simulink model "full_system_phase_control_dq0_discrete_quantized"  (R2015b)
settings: Solver=VariableStepAuto  StartTime=0.0  StopTime=6  FixedStep=1  RelTol=1e-2
values from neighbouring files (symbols this model uses):
  ad = cos(8*pi/256*n1+offset)    [Parameters.m]
  aq = -sin(8*pi/256*n1+offset)    [Parameters.m]
  bd = cos(8*pi/256*n1+offset-2/3*pi)    [Parameters.m]
  bq = -sin(8*pi/256*n1+offset-2/3*pi)    [Parameters.m]
  c_drag = -1/2*1.225*.804*.6    (= -0.29547)    [Parameters.m]
  cd = cos(8*pi/256*n1+offset+2/3*pi)    [Parameters.m]
  cq = -sin(8*pi/256*n1+offset+2/3*pi)    [Parameters.m]
  G1 = 12    [Parameters.m]
  G2 = 50    [Parameters.m]
  Ki = (3*alpha^2-((Kp*Kv)/(2*J_pro)-(Kv*R)/(J_pro*L)-(3*Kt^2)/(2*J_pro*L)))*L    (= 1.75664037993)    [Parameters.m]
  Kp = (3*alpha-Kv/J_pro-(R/(2*L)))*L    (= 0.0111498579282)    [Parameters.m]
  Kt = .07329    (= 0.07329)    [Parameters.m]
  L = 4e-5    (= 4e-05)    [Parameters.m]
  N = 4    [Parameters.m]
  n1 = 0:255    [Parameters.m]
  n2 = -1:.01:1    [Parameters.m]
  offset = 0    [Parameters.m]
  r = 11*.0254/2    (= 0.1397)    [Parameters.m]
  T = 1/10000    (= 0.0001)    [Parameters.m]
  third_phase = sin(3*asin(n2))    [Parameters.m]
undefined symbols (not defined in the file or in its folder): DiscIntNeverNeededParam, sigbuilder_block
libraries: fl_lib x19, nesl_utility x11, pe_lib x2, simulink x2, powerlib_meascontrol x1
settings Model: Creator=Martin Andersen  LastModifiedBy=Martin Andersen
settings SolverCC: AlgebraicLoopSolver=LineSearch

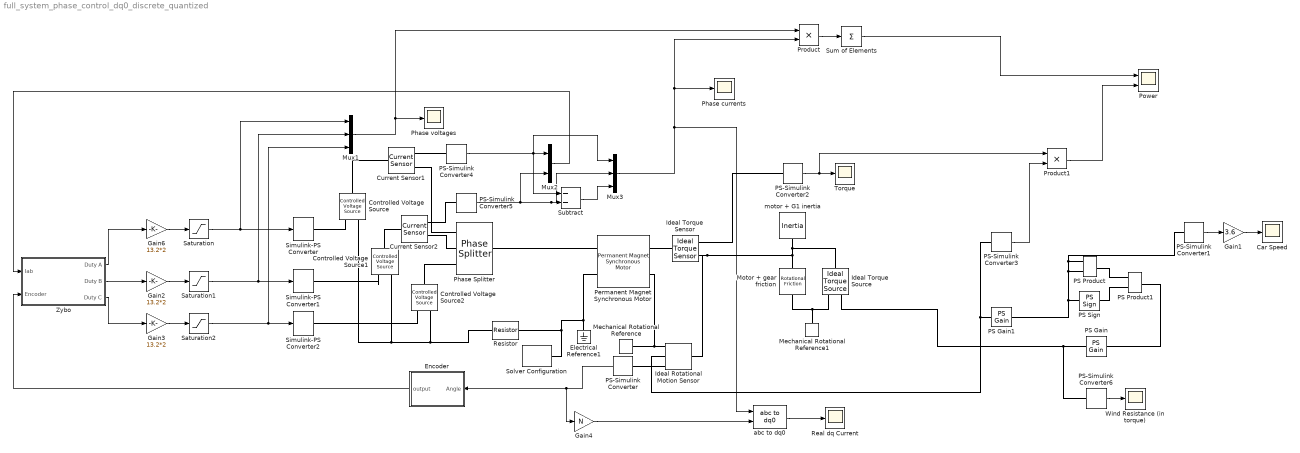
== system full_system_phase_control_dq0_discrete_quantized ==
  Car Speed : Scope
  Controlled Voltage Source : fl_lib/Electrical/Electrical Sources/Controlled Voltage Source
  Controlled Voltage Source1 : fl_lib/Electrical/Electrical Sources/Controlled Voltage Source
  Controlled Voltage Source2 : fl_lib/Electrical/Electrical Sources/Controlled Voltage Source
  Current Sensor1 : fl_lib/Electrical/Electrical Sensors/Current Sensor
  Current Sensor2 : fl_lib/Electrical/Electrical Sensors/Current Sensor
  Electrical Reference1 : fl_lib/Electrical/Electrical Elements/Electrical Reference
  Encoder : Subsystem
  Gain1 : Gain  Gain=3.6
  Gain2 : Gain  Gain=13.2*2
  Gain3 : Gain  Gain=13.2*2
  Gain4 : Gain  Gain=N
  Gain6 : Gain  Gain=13.2*2
  Ideal Rotational Motion Sensor : fl_lib/Mechanical/Mechanical Sensors/Ideal Rotational Motion Sensor  offset=0 rad
  Ideal Torque Sensor : fl_lib/Mechanical/Mechanical Sensors/Ideal Torque Sensor
  Ideal Torque Source : fl_lib/Mechanical/Mechanical Sources/Ideal Torque Source
  Mechanical Rotational Reference : fl_lib/Mechanical/Rotational Elements/Mechanical Rotational Reference
  Mechanical Rotational Reference1 : fl_lib/Mechanical/Rotational Elements/Mechanical Rotational Reference
  Motor + gear friction : fl_lib/Mechanical/Rotational Elements/Rotational Friction  brkwy_trq=.5 N*m  Col_trq=.2 N*m  visc_coef=0.0001 N*m/(rad/s)  trans_coef=10 s/rad  vel_thr=1e-4 rad/s  w_specify=off  w_priority=None  w=0 rad/s  t_specify=off  t_priority=None  t=0 N*m
  Mux1 : Mux  Inputs=3
  Mux2 : Mux  Inputs=2
  Mux3 : Mux  Inputs=3
  PS Gain : fl_lib/Physical Signals/Functions/PS Gain  gain=c_drag*G1/G2*r
  PS Gain1 : fl_lib/Physical Signals/Functions/PS Gain  gain=G1/G2*r
  PS Product : fl_lib/Physical Signals/Functions/PS Product
  PS Product1 : fl_lib/Physical Signals/Functions/PS Product
  PS Sign : fl_lib/Physical Signals/Nonlinear Operators/PS Sign
  PS-Simulink Converter{,1..6} (7 alike) : nesl_utility/PS-Simulink Converter  PhysicalDomain=network_engine_domain  SubClassName=ps_output  LeftPortType=input  RightPortType=output  PseudoPeriodic=off  Frequencies=[]  Unit=1  AffineConversion=off
  Permanent Magnet Synchronous Motor : pe_lib/Machines/Permanent Magnet Rotor/Permanent Magnet Synchronous Motor  nPolePairs=N  pm_flux_linkage=Kt/N Wb  stator_param=1  Ld=L H  Lq=L H  L0=L H  Ls=L H  Lm=0 H  Ms=L/10 H  Rs=R Ohm  initial_currents=[0, 0, 0] A  axes_param=2  angular_position0=0 rad  rotor_offset=- pi / 2 rad  shift_3ph=[nan, nan, nan] rad  sqrt2OverSqrt3=nan  oneOverSqrt2=nan  twoPiOver3=nan  Lmin=1e-9 H
  Phase Splitter : pe_lib/Connections/Phase Splitter
  Phase currents : Scope
  Phase voltages : Scope
  Power : Scope  NumInputPorts=2
  Product : Product
  Product1 : Product
  Real dq Current : Scope
  Resistor : fl_lib/Electrical/Electrical Elements/Resistor  R=1e9 Ohm  i_specify=off  i_priority=None  i=0 A  v_specify=off  v_priority=None  v=0 V
  Saturation : Saturate  UpperLimit=13.2*2  LowerLimit=-13.2*2
  Saturation1 : Saturate  UpperLimit=13.2*2  LowerLimit=-13.2*2
  Saturation2 : Saturate  UpperLimit=13.2*2  LowerLimit=-13.2*2
  Simulink-PS Converter : nesl_utility/Simulink-PS Converter  PhysicalDomain=network_engine_domain  SubClassName=ps_input  LeftPortType=input  RightPortType=output  PseudoPeriodic=off  Frequencies=[]  NoiseDistribution=none  NoiseParameters=[]  Unit=1  AffineConversion=off  InputFiltering=off  SimscapeFilterOrder=1  InputFilterTimeConstant=0.001  UdotUserProvided=1
  Simulink-PS Converter1 : nesl_utility/Simulink-PS Converter  PhysicalDomain=network_engine_domain  SubClassName=ps_input  LeftPortType=input  RightPortType=output  PseudoPeriodic=off  Frequencies=[]  NoiseDistribution=none  NoiseParameters=[]  Unit=1  AffineConversion=off  InputFiltering=off  SimscapeFilterOrder=1  InputFilterTimeConstant=0.001  UdotUserProvided=1
  Simulink-PS Converter2 : nesl_utility/Simulink-PS Converter  PhysicalDomain=network_engine_domain  SubClassName=ps_input  LeftPortType=input  RightPortType=output  PseudoPeriodic=off  Frequencies=[]  NoiseDistribution=none  NoiseParameters=[]  Unit=1  AffineConversion=off  InputFiltering=off  SimscapeFilterOrder=1  InputFilterTimeConstant=0.001  UdotUserProvided=1
  Solver Configuration : nesl_utility/Solver Configuration  PhysicalDomain=network_engine_domain  SubClassName=solver  LeftPortType=input  RightPortType=generic  Accelerate=off  Tones=[]  Harmonics=[]  SimulateNoise=off  Profile=off  UseLocalSampling=off  EnableSwitchedLinearOptims=on  FrequencyDomain=off  UseCCode=off  RelTol=0.001  AbsTol=1e-06  MinStep=1e-09  ToWorkspace=off  RevertToSquareIcSolve=off  NumHomotopyIterations=100  PhasorMode=off  PhasorModeNumHarmonics=1  DoDC=off  ResidualTolerance=1e-09  UseLocalSolver=off  LocalSolverChoice=NE_BACKWARD_EULER_ADVANCER  LocalSolverSampleTime=0.001  DoFixedCost=off  MaxNonlinIter=3  MaxModeIter=2  LinearAlgebra=Sparse  DelaysMemoryBudget=1024  AutomaticFiltering=on  FilteringTimeConstant=0.001
  Subtract : Sum  Inputs=--
  Sum of Elements : Sum  Inputs=+
  Torque : Scope
  Wind Resistance (in torque) : Scope
  Zybo : Subsystem
  abc to dq0 : powerlib_meascontrol/Transformations/abc to dq0  Alignment=Aligned with phase A axis
  motor + G1 inertia : fl_lib/Mechanical/Rotational Elements/Inertia  inertia=J_pro kg*m^2  w_specify=off  w_priority=None  w=0 rad/s  t_specify=off  t_priority=None  t=0 N*m
  wires:
  PS-Simulink Converter1/1 -> Gain1/1
  Gain1/1 -> Car Speed/1
  PS-Simulink Converter4/1 -> Subtract/1, Mux3/1, Mux2/1
  PS-Simulink Converter5/1 -> Mux3/2, Subtract/2, Mux2/2
  PS-Simulink Converter6/1 -> Wind Resistance (in torque)/1
  Mux1/1 -> Product/1, Phase voltages/1
  Mux2/1 -> Zybo/1(Iab)
  PS-Simulink Converter2/1 -> Product1/1, Torque/1
  Product/1 -> Sum of Elements/1
  Sum of Elements/1 -> Power/1
  PS-Simulink Converter3/1 -> Product1/2
  Product1/1 -> Power/2
  Zybo/1(Duty A) -> Gain6/1
  PS-Simulink Converter/1 -> Gain4/1, Encoder/1(Angle)
  Encoder/1(output) -> Zybo/2(Encoder)
  Gain6/1 -> Saturation/1
  Gain2/1 -> Saturation1/1
  Gain3/1 -> Saturation2/1
  Saturation/1 -> Mux1/1, Simulink-PS Converter/1
  Saturation1/1 -> Mux1/2, Simulink-PS Converter1/1
  Zybo/2(Duty B) -> Gain2/1
  Zybo/3(Duty C) -> Gain3/1
  Saturation2/1 -> Mux1/3, Simulink-PS Converter2/1
  Subtract/1 -> Mux3/3
  Mux3/1 -> abc to dq0/1, Phase currents/1, Product/2
  Gain4/1 -> abc to dq0/2
  abc to dq0/1 -> Real dq Current/1
  connections:
  Permanent Magnet Synchronous Motor/LConn2 -- Resistor/RConn1 -- Solver Configuration/RConn1 -- Electrical Reference1/LConn1
  Ideal Rotational Motion Sensor/RConn1 -- Mechanical Rotational Reference/LConn1 -- Permanent Magnet Synchronous Motor/RConn2
  PS Sign/LConn1 -- PS-Simulink Converter1/LConn1 -- PS Product/LConn1 -- PS Product/LConn2 -- PS Gain1/RConn1
  PS Product1/LConn2 -- PS Sign/RConn1
  PS Product1/LConn1 -- PS Product/RConn1
  PS Gain/LConn1 -- PS Product1/RConn1
  PS-Simulink Converter6/LConn1 -- Ideal Torque Source/RConn1 -- PS Gain/RConn1
  PS-Simulink Converter/LConn1 -- Ideal Rotational Motion Sensor/RConn3
  Controlled Voltage Source/RConn1 -- Simulink-PS Converter/RConn1
  Controlled Voltage Source1/RConn1 -- Simulink-PS Converter1/RConn1
  Controlled Voltage Source2/RConn1 -- Simulink-PS Converter2/RConn1
  Controlled Voltage Source2/LConn1 -- Phase Splitter/RConn3
  Controlled Voltage Source1/RConn2 -- Controlled Voltage Source/RConn2 -- Resistor/LConn1 -- Controlled Voltage Source2/RConn2
  Phase Splitter/LConn1 -- Permanent Magnet Synchronous Motor/LConn1
  Current Sensor1/LConn1 -- Controlled Voltage Source/LConn1
  Current Sensor1/RConn2 -- Phase Splitter/RConn1
  Current Sensor2/LConn1 -- Controlled Voltage Source1/LConn1
  Current Sensor2/RConn2 -- Phase Splitter/RConn2
  PS-Simulink Converter4/LConn1 -- Current Sensor1/RConn1
  Current Sensor2/RConn1 -- PS-Simulink Converter5/LConn1
  Mechanical Rotational Reference1/LConn1 -- Ideal Torque Source/RConn2 -- Motor + gear friction/RConn1
  PS Gain1/LConn1 -- Ideal Rotational Motion Sensor/RConn2 -- PS-Simulink Converter3/LConn1
  motor + G1 inertia/LConn1 -- Ideal Rotational Motion Sensor/LConn1 -- Ideal Torque Sensor/RConn1 -- Motor + gear friction/LConn1 -- Ideal Torque Source/LConn1
  PS-Simulink Converter2/LConn1 -- Ideal Torque Sensor/RConn2
  Ideal Torque Sensor/LConn1 -- Permanent Magnet Synchronous Motor/RConn1

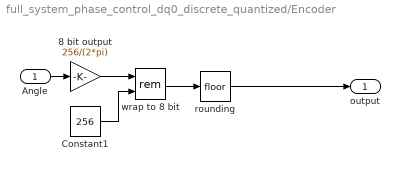
== system full_system_phase_control_dq0_discrete_quantized/Encoder ==
  Angle : Inport
  8 bit output : Gain  Gain=256/(2*pi)
  Constant1 : Constant  Value=256
  rounding : Rounding
  wrap to 8 bit : Math  Operator=rem  SaturateOnIntegerOverflow=on
  output : Outport
  wires:
  wrap to 8 bit/1 -> rounding/1
  Constant1/1 -> wrap to 8 bit/2
  8 bit output/1 -> wrap to 8 bit/1
  Angle/1 -> 8 bit output/1
  rounding/1 -> output/1

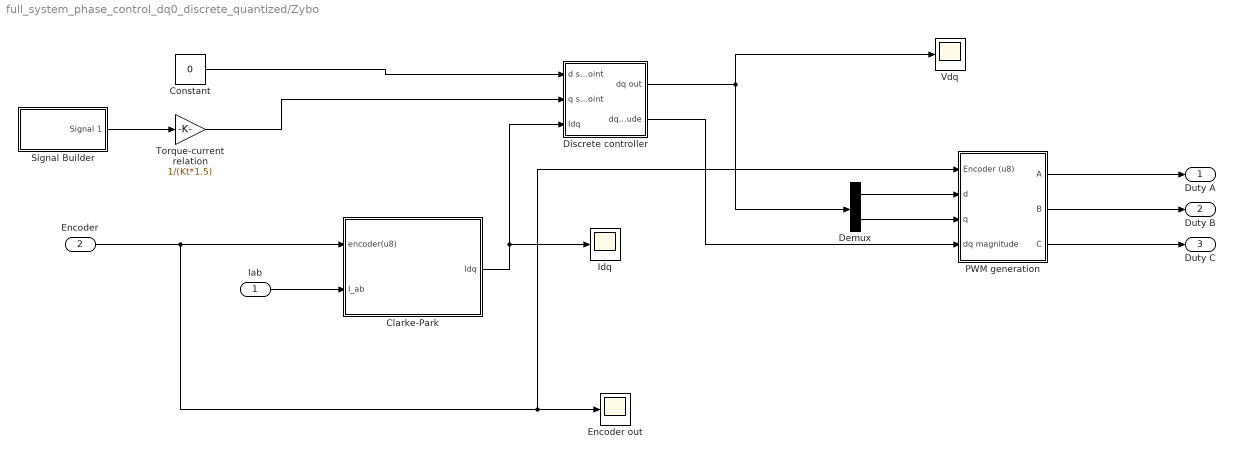
== system full_system_phase_control_dq0_discrete_quantized/Zybo ==
  Iab : Inport
  Encoder : Inport  Port=2
  Clarke-Park : Subsystem  SystemSampleTime=T
  Constant : Constant  Value=0
  Demux : Demux  Outputs=2
  Discrete controller : Subsystem  TreatAsAtomicUnit=on  SystemSampleTime=T
  Encoder out : Scope
  Idq : Scope
  PWM generation : Subsystem
  Signal Builder : Subsystem  Tag=STV Subsys  LoadFcn=sigbuilder_block('load',[298.8 170.4 550.8 400.2 ]);  StartFcn=sigbuilder_block('start');  StopFcn=sigbuilder_block('stop');  ClipboardFcn=sigbuilder_block('clipboard');  mask(Sigbuilder block){}
      mask help: Simulink:masks:SigbuilderBlock_MD
      mask init:
      | if ~strcmp(get_param(bdroot(gcbh),'SimulationStatus'),'stopped') tuvar = sigbuilder_block('maskInit'); end
      settings: CopyFcn=sigbuilder_block('copy');  DeleteFcn=sigbuilder_block('delete');  ModelCloseFcn=sigbuilder_block('modelClose');  PreSaveFcn=sigbuilder_block('preSave');  PauseFcn=sigbuilder_block('pause');  ContinueFcn=sigbuilder_block('continue');  NameChangeFcn=sigbuilder_block('namechange');  OpenFcn=sigbuilder_block('open',[298.8 170.4 550.8 400.2 ]);  CloseFcn=sigbuilder_block('close');
      mask Display: plot(0, 0, 100, 100,[2, 2, 32, 32, 2], [68, 8, 8, 68, 68],[32, 2], [38, 38], [32, 19, 2],[53, 60, 44], [32, 17, 17, 2],[16, 16, 31, 31]);txt = getActiveGroup(gcbh);text(2, 100, txt,'verticalAlignment', 'top');
  Torque-current relation : Gain  Gain=1/(Kt*1.5)
  Vdq : Scope
  Duty A : Outport
  Duty B : Outport  Port=2
  Duty C : Outport  Port=3
  wires:
  Demux/1 -> PWM generation/2(d)
  Discrete controller/2(dq magnitude) -> PWM generation/4(dq magnitude)
  Demux/2 -> PWM generation/3(q)
  PWM generation/3(C) -> Duty C/1
  PWM generation/1(A) -> Duty A/1
  PWM generation/2(B) -> Duty B/1
  Constant/1 -> Discrete controller/1(d setpoint)
  Torque-current relation/1 -> Discrete controller/2(q setpoint)
  Signal Builder/1(Signal 1) -> Torque-current relation/1
  Discrete controller/1(dq out) -> Vdq/1, Demux/1
  Iab/1 -> Clarke-Park/2(I_ab)
  Clarke-Park/1(Idq) -> Idq/1, Discrete controller/3(Idq)
  Encoder/1 -> Clarke-Park/1(encoder(u8)), PWM generation/1(Encoder (u8)), Encoder out/1

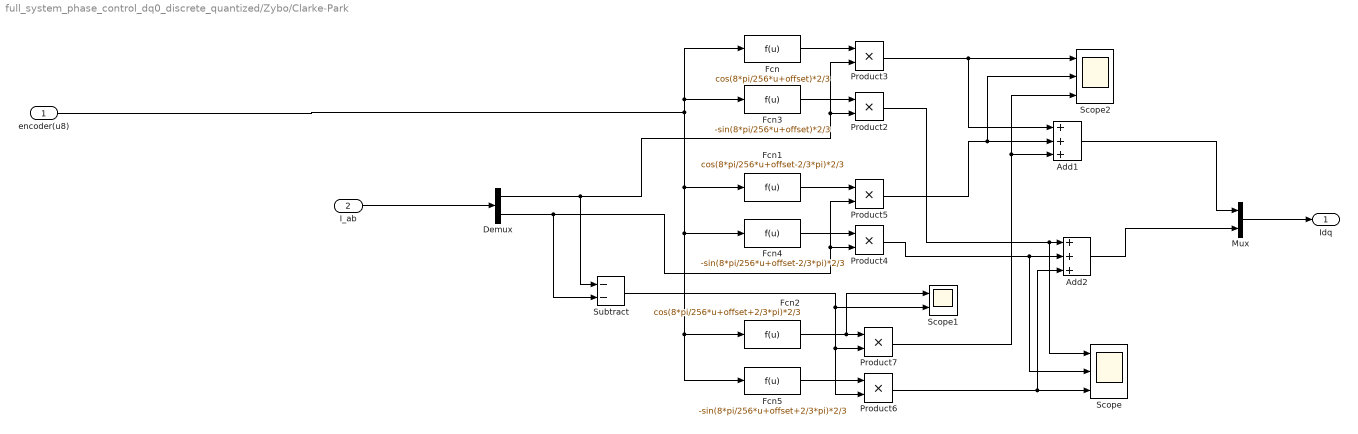
== system full_system_phase_control_dq0_discrete_quantized/Zybo/Clarke-Park ==
  encoder(u8) : Inport
  I_ab : Inport  Port=2
  Add1 : Sum  Inputs=+++
  Add2 : Sum  Inputs=+++
  Demux : Demux  Outputs=2
  Fcn : Fcn  Expr=cos(8*pi/256*u+offset)*2/3
  Fcn1 : Fcn  Expr=cos(8*pi/256*u+offset-2/3*pi)*2/3
  Fcn2 : Fcn  Expr=cos(8*pi/256*u+offset+2/3*pi)*2/3
  Fcn3 : Fcn  Expr=-sin(8*pi/256*u+offset)*2/3
  Fcn4 : Fcn  Expr=-sin(8*pi/256*u+offset-2/3*pi)*2/3
  Fcn5 : Fcn  Expr=-sin(8*pi/256*u+offset+2/3*pi)*2/3
  Mux : Mux  Inputs=2
  Product{2..7} (6 alike) : Product
  Scope : Scope  NumInputPorts=3
  Scope1 : Scope  NumInputPorts=2
  Scope2 : Scope  NumInputPorts=3
  Subtract : Sum  Inputs=--
  Idq : Outport
  wires:
  Add2/1 -> Mux/2
  Fcn/1 -> Product3/1
  Fcn5/1 -> Product6/1
  Demux/1 -> Product2/2, Product3/2, Subtract/1
  Fcn4/1 -> Product4/1
  I_ab/1 -> Demux/1
  Subtract/1 -> Product6/2, Product7/2, Scope1/2
  Product6/1 -> Scope/3, Add2/3
  Product4/1 -> Scope/2, Add2/2
  Fcn3/1 -> Product2/1
  Product5/1 -> Scope2/2, Add1/2
  Fcn1/1 -> Product5/1
  Demux/2 -> Subtract/2, Product5/2, Product4/2
  Fcn2/1 -> Scope1/1, Product7/1
  Product3/1 -> Scope2/1, Add1/1
  Product2/1 -> Scope/1, Add2/1
  Product7/1 -> Scope2/3, Add1/3
  encoder(u8)/1 -> Fcn1/1, Fcn4/1, Fcn5/1, Fcn2/1, Fcn3/1, Fcn/1
  Mux/1 -> Idq/1
  Add1/1 -> Mux/1

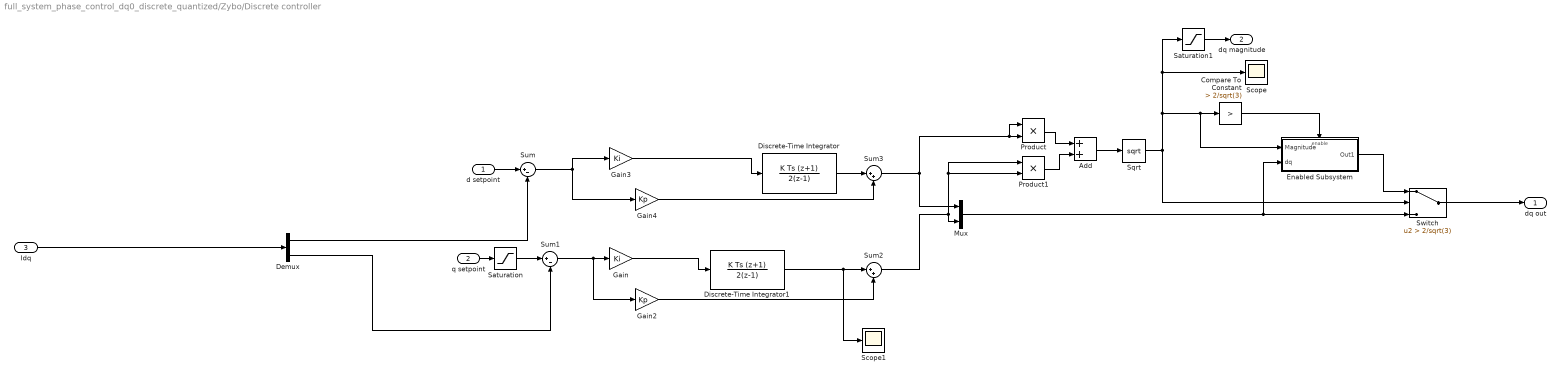
== system full_system_phase_control_dq0_discrete_quantized/Zybo/Discrete controller ==
  d setpoint : Inport
  q setpoint : Inport  Port=2
  Idq : Inport  Port=3
  Add : Sum
  Compare To Constant : simulink/Logic and Bit Operations/Compare To Constant  relop=>  const=2/sqrt(3)  OutDataTypeStr=boolean
  Demux : Demux  Outputs=2
  Discrete-Time Integrator : DiscreteIntegrator  IntegratorMethod=Integration: Trapezoidal  InitialConditionSetting=State (most efficient)  SampleTime=T  LimitOutput=on  UpperSaturationLimit=2/sqrt(3)  LowerSaturationLimit=-2/sqrt(3)  ICPrevOutput=DiscIntNeverNeededParam  ICPrevScaledInput=DiscIntNeverNeededParam
  Discrete-Time Integrator1 : DiscreteIntegrator  IntegratorMethod=Integration: Trapezoidal  InitialConditionSetting=State (most efficient)  SampleTime=T  LimitOutput=on  UpperSaturationLimit=2/sqrt(3)  LowerSaturationLimit=-2/sqrt(3)  ICPrevOutput=DiscIntNeverNeededParam  ICPrevScaledInput=DiscIntNeverNeededParam
  Enabled Subsystem : Subsystem  TreatAsAtomicUnit=on
  Gain : Gain  Gain=Ki
  Gain2 : Gain  Gain=Kp
  Gain3 : Gain  Gain=Ki
  Gain4 : Gain  Gain=Kp
  Mux : Mux  Inputs=2
  Product : Product
  Product1 : Product
  Saturation : Saturate  UpperLimit=300
  Saturation1 : Saturate  UpperLimit=2/sqrt(3)
  Scope : Scope
  Scope1 : Scope
  Sqrt : Sqrt  SaturateOnIntegerOverflow=on
  Sum : Sum  Inputs=|+-
  Sum1 : Sum  Inputs=|+-
  Sum2 : Sum  Inputs=|++
  Sum3 : Sum  Inputs=|++
  Switch : Switch  Criteria=u2 > Threshold  Threshold=2/sqrt(3)
  dq out : Outport
  dq magnitude : Outport  Port=2
  wires:
  Sum1/1 -> Gain2/1, Gain/1
  Gain4/1 -> Sum3/2
  Sum/1 -> Gain4/1, Gain3/1
  Gain2/1 -> Sum2/2
  Gain/1 -> Discrete-Time Integrator1/1
  Gain3/1 -> Discrete-Time Integrator/1
  Discrete-Time Integrator/1 -> Sum3/1
  Mux/1 -> Enabled Subsystem/2(dq), Switch/3
  Discrete-Time Integrator1/1 -> Scope1/1, Sum2/1
  Sum3/1 -> Mux/1, Product/1, Product/2
  Sum2/1 -> Product1/2, Product1/1, Mux/2
  Product/1 -> Add/1
  Product1/1 -> Add/2
  Add/1 -> Sqrt/1
  q setpoint/1 -> Saturation/1
  d setpoint/1 -> Sum/1
  Saturation/1 -> Sum1/1
  Switch/1 -> dq out/1
  Compare To Constant/1 -> Enabled Subsystem/Enable
  Enabled Subsystem/1(Out1) -> Switch/1
  Sqrt/1 -> Switch/2, Enabled Subsystem/1(Magnitude), Compare To Constant/1, Saturation1/1, Scope/1
  Idq/1 -> Demux/1
  Demux/1 -> Sum/2
  Demux/2 -> Sum1/2
  Saturation1/1 -> dq magnitude/1

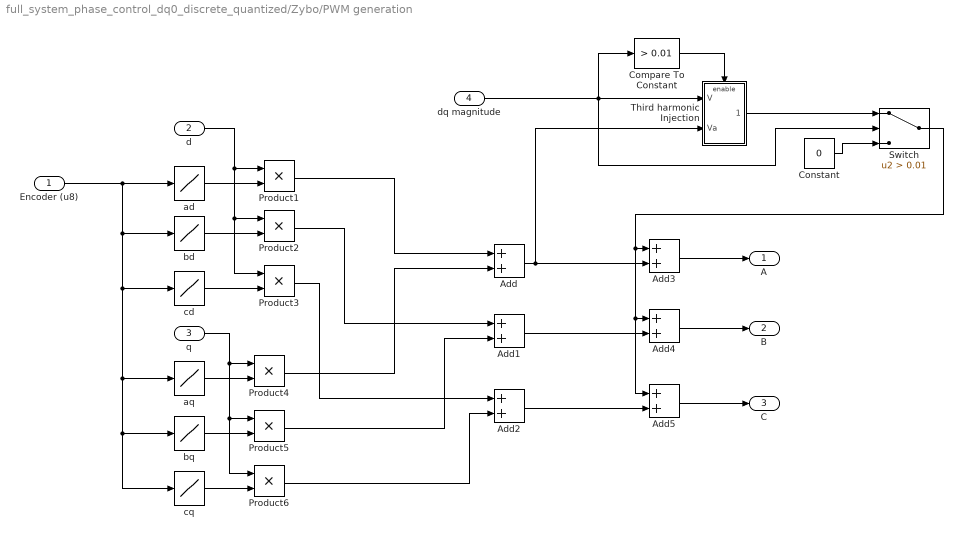
== system full_system_phase_control_dq0_discrete_quantized/Zybo/PWM generation ==
  Encoder (u8) : Inport
  d : Inport  Port=2
  q : Inport  Port=3
  dq magnitude : Inport  Port=4
  Add{,1..5} (6 alike) : Sum
  Compare To Constant : simulink/Logic and Bit Operations/Compare To Constant  relop=>  const=0.01  OutDataTypeStr=boolean
  Constant : Constant  Value=0
  Product{1..6} (6 alike) : Product
  Switch : Switch  Criteria=u2 > Threshold  Threshold=0.01
  Third harmonic Injection : Subsystem
  ad : Lookup_n-D  NumberOfTableDimensions=1  BreakpointsForDimension1=n1  IndexSearchMethod=Linear search  Table=ad  InterpMethod=Nearest  InternalRulePriority=Speed  RndMeth=Simplest  InputSameDT=on
  aq : Lookup_n-D  NumberOfTableDimensions=1  BreakpointsForDimension1=n1  Table=aq  InterpMethod=Nearest  InternalRulePriority=Speed  RndMeth=Simplest  InputSameDT=on
  bd : Lookup_n-D  NumberOfTableDimensions=1  BreakpointsForDimension1=n1  Table=bd  InterpMethod=Nearest  InternalRulePriority=Speed  RndMeth=Simplest  InputSameDT=on
  bq : Lookup_n-D  NumberOfTableDimensions=1  BreakpointsForDimension1=n1  Table=bq  InterpMethod=Nearest  InternalRulePriority=Speed  RndMeth=Simplest  InputSameDT=on
  cd : Lookup_n-D  NumberOfTableDimensions=1  BreakpointsForDimension1=n1  Table=cd  InterpMethod=Nearest  InternalRulePriority=Speed  RndMeth=Simplest  InputSameDT=on
  cq : Lookup_n-D  NumberOfTableDimensions=1  BreakpointsForDimension1=n1  Table=cq  InterpMethod=Nearest  InternalRulePriority=Speed  RndMeth=Simplest  InputSameDT=on
  A : Outport
  B : Outport  Port=2
  C : Outport  Port=3
  wires:
  Encoder (u8)/1 -> cq/1, bq/1, aq/1, cd/1, bd/1, ad/1
  cd/1 -> Product3/2
  bd/1 -> Product2/2
  ad/1 -> Product1/2
  d/1 -> Product3/1, Product2/1, Product1/1
  bq/1 -> Product5/2
  cq/1 -> Product6/2
  aq/1 -> Product4/2
  q/1 -> Product6/1, Product5/1, Product4/1
  Add5/1 -> C/1
  Add4/1 -> B/1
  Add3/1 -> A/1
  Add1/1 -> Add4/2
  Add/1 -> Third harmonic Injection/2(Va), Add3/2
  Add2/1 -> Add5/2
  Product1/1 -> Add/1
  Product4/1 -> Add/2
  Product2/1 -> Add1/1
  Product5/1 -> Add1/2
  Product3/1 -> Add2/1
  Product6/1 -> Add2/2
  dq magnitude/1 -> Switch/2, Compare To Constant/1, Third harmonic Injection/1(V)
  Switch/1 -> Add5/1, Add4/1, Add3/1
  Third harmonic Injection/1(Third Harmonic) -> Switch/1
  Compare To Constant/1 -> Third harmonic Injection/Enable
  Constant/1 -> Switch/3

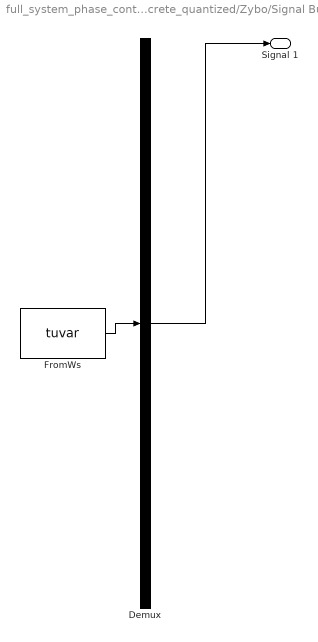
== system full_system_phase_control_dq0_discrete_quantized/Zybo/Signal Builder ==
  Demux : Demux  Tag=STV Demux  Outputs=1
  FromWs : FromWorkspace  Tag=STV FromWs  VariableName=tuvar  SampleTime=0
      SigBuilderData=|
      | common.afterFinalStr = 'Extrapolate'
      | common.sampleTime = 0
      | dataSet.timeRange = [0 10]
      | dataSet.name = 'Group 1'
      | sbobj.Groups.Name = 'Group 1'
      | sbobj.Groups.Signals.Name = 'Signal 1'
      | sbobj.Groups.Signals.XData = [0 0.32 5.5 5.5 10]
      | sbobj.Groups.Signals.YData = [0 40.6 40.6 0 0]
  Signal 1 : Outport  Tag=STV Outport
  wires:
  Demux/1 -> Signal 1/1
  FromWs/1 -> Demux/1

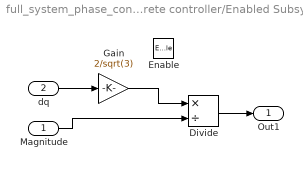
== system full_system_phase_control_dq0_discrete_quantized/Zybo/Discrete controller/Enabled Subsystem ==
  Magnitude : Inport
  dq : Inport  Port=2
  Enable : EnablePort
  Divide : Product  Inputs=*/
  Gain : Gain  Gain=2/sqrt(3)
  Out1 : Outport
  wires:
  dq/1 -> Gain/1
  Magnitude/1 -> Divide/2
  Divide/1 -> Out1/1
  Gain/1 -> Divide/1

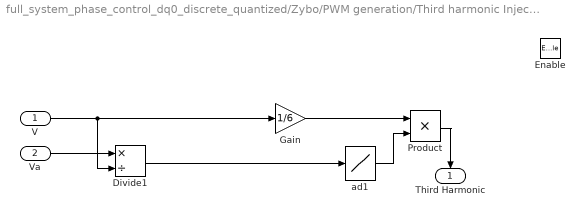
== system full_system_phase_control_dq0_discrete_quantized/Zybo/PWM generation/Third harmonic Injection ==
  V : Inport
  Va : Inport  Port=2
  Enable : EnablePort
  Divide1 : Product  Inputs=*/
  Gain : Gain  Gain=1/6
  Product : Product
  ad1 : Lookup_n-D  NumberOfTableDimensions=1  BreakpointsForDimension1=n2  Table=third_phase  InterpMethod=Nearest  InternalRulePriority=Speed  RndMeth=Simplest  InputSameDT=on
  Third Harmonic : Outport
  wires:
  V/1 -> Divide1/2, Gain/1
  Gain/1 -> Product/1
  ad1/1 -> Product/2
  Product/1 -> Third Harmonic/1
  Va/1 -> Divide1/1
  Divide1/1 -> ad1/1
